simulink model "HybridMPC"  (R2024b)
settings: Solver=VariableStepAuto  StartTime=0.0  StopTime=50  RelTol=1e-3
undefined symbols (not defined in the file or in its folder): A1, A2, B1, B2, C
libraries: mpclib x1
settings Model: Creator=Reza Shahriari  LastModifiedBy=Reza Shahriari

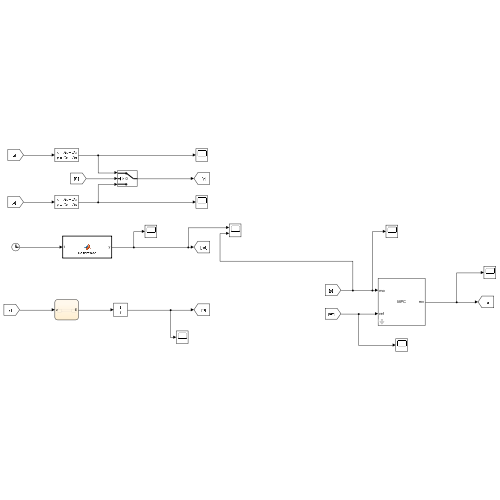
[thumbnail: Simulink's stored preview of the top-level diagram]
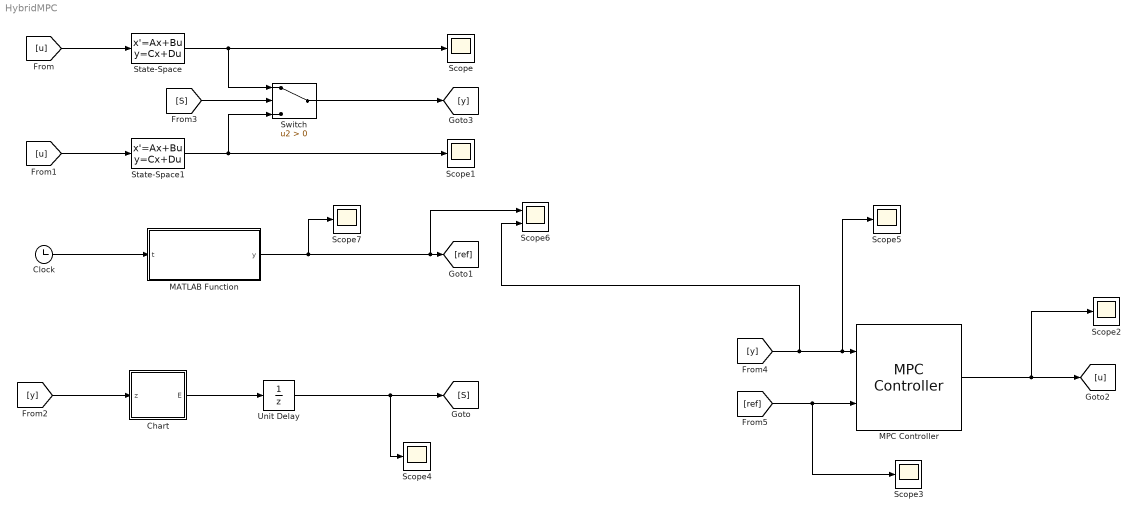
== system HybridMPC ==
  Chart : Stateflow chart  TreatAsAtomicUnit=on
  Clock : Clock
  MATLAB Function : MATLAB Function  TreatAsAtomicUnit=on
  MPC Controller : mpclib/MPC Controller  SCDEnableBlockLinearizationSpecification=on  mpcobj=mpc1  is_multiple=0  enable_value=0  return_u0=off  updateMPCinCallerWorkspace=on  md_inport=off  mv_inport=off  uref_inport=off  return_cost=off  return_mvseq=off  return_qpstatus=off  return_xseq=off  return_state=off  return_ovseq=off  state_inport=off  umin_inport=off  umax_inport=off  ymin_inport=off  ymax_inport=off  cc_inport=off  ywt_inport=off  uwt_inport=off  duwt_inport=off  rhoeps_inport=off  pm_inport=off  MaximumP=10  HorizonChoice=FixedHorizon  n_ts=0.01  n_p=20  n_mv=1  n_md=0  n_ud=0  n_mo=1  n_uo=0  BlockDataType=double  SampleTimeInherited=off  switch_inport=off
  Scope{,1..5,7} (7 alike) : Scope
  Scope6 : Scope  NumInputPorts=2
  State-Space : StateSpace  A=A1  B=B1  C=C  D=0  InitialCondition=[0.5;0]
  State-Space1 : StateSpace  A=A2  B=B2  C=C  D=0  InitialCondition=[0.5;0]
  Switch : Switch  Criteria=u2 > Threshold  SaturateOnIntegerOverflow=off  InputSameDT=off
  Unit Delay : UnitDelay  SampleTime=-1  HasFrameUpgradeWarning=on
  wires:
  State-Space/1 -> Switch/1, Scope/1
  State-Space1/1 -> Scope1/1, Switch/3
  [u] -> State-Space/1
  [u] -> State-Space1/1
  Clock/1 -> MATLAB Function/1(t)
  [y] -> Chart/1(z)
  Chart/1(E) -> Unit Delay/1
  Unit Delay/1 -> Scope4/1, [S]
  MATLAB Function/1(y) -> Scope7/1, Scope6/1, [ref]
  [y] -> Scope6/2, Scope5/1, MPC Controller/1
  [ref] -> Scope3/1, MPC Controller/2
  MPC Controller/1 -> Scope2/1, [u]
  [S] -> Switch/2
  Switch/1 -> [y]

== matlab function HybridMPC/MATLAB Function ==
  data: t input; y output
function y = Reference(t)

y = 20*sin((2*pi*t)/20);

== stateflow chart HybridMPC/Chart ==
  state MODE1
    en: E=0
  state MODE2
    en:E=1
  (default) -> MODE1
  MODE1 -> MODE2 : [z>5]
  MODE2 -> MODE1 : [z<-5]
  data: z input; E output
